simulink model "kalmannonlinear"  (R2019b)
settings: Solver=VariableStepAuto  StartTime=0.0  StopTime=10.0  RelTol=1e-3
libraries: sharedTrackingLibrary x2
settings Model: Creator=Bekircan Keceoglu  LastModifiedBy=Bekircan Keceoglu

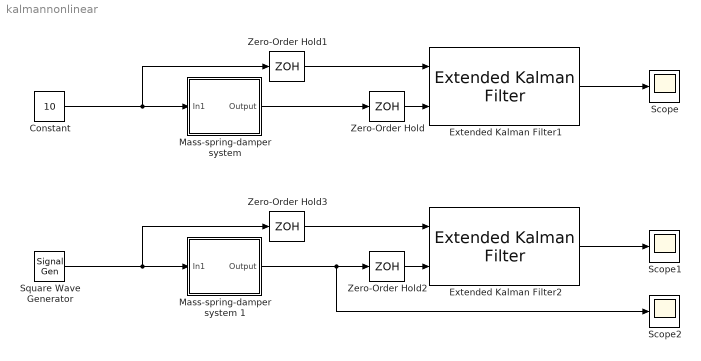
== system kalmannonlinear ==
  Constant : Constant  Value=10
  Extended Kalman Filter1 : sharedTrackingLibrary/Extended Kalman Filter  StateTransitionFcn=myStateTransitionFcn  HasStateTransitionJacobianFcn=off  HasAdditiveProcessNoise=Additive  ProcessNoise=1  HasTimeVaryingProcessNoise=off  HasStateTransitionFcnExtraArgument=1  InitialState=[0 0]  InitialStateCovariance=1  MeasurementFcn1=myMeasurementFcn  HasMeasurementJacobianFcn1=off  HasMeasurementEnablePort1=off  HasAdditiveMeasurementNoise1=Additive  MeasurementNoise1=1  HasTimeVaryingMeasurementNoise1=off  HasMeasurementFcnExtraArgument1=0  MeasurementFcn2=myMeasurementFcn  HasMeasurementJacobianFcn2=off  HasMeasurementEnablePort2=off  HasAdditiveMeasurementNoise2=Additive  MeasurementNoise2=1  HasTimeVaryingMeasurementNoise2=off  HasMeasurementFcnExtraArgument2=0  MeasurementFcn3=myMeasurementFcn  HasMeasurementJacobianFcn3=off  HasMeasurementEnablePort3=off  HasAdditiveMeasurementNoise3=Additive  MeasurementNoise3=1  HasTimeVaryingMeasurementNoise3=off  HasMeasurementFcnExtraArgument3=0  MeasurementFcn4=myMeasurementFcn  HasMeasurementJacobianFcn4=off  HasMeasurementEnablePort4=off  HasAdditiveMeasurementNoise4=Additive  MeasurementNoise4=1  HasTimeVaryingMeasurementNoise4=off  HasMeasurementFcnExtraArgument4=0  MeasurementFcn5=myMeasurementFcn  HasMeasurementJacobianFcn5=off  HasMeasurementEnablePort5=off  HasAdditiveMeasurementNoise5=Additive  MeasurementNoise5=1  HasTimeVaryingMeasurementNoise5=off  HasMeasurementFcnExtraArgument5=0  EnableMultirate=off  StateTransitionFcnSampleTime=1  MeasurementFcn1SampleTime=1  MeasurementFcn2SampleTime=1  MeasurementFcn3SampleTime=1  MeasurementFcn4SampleTime=1  MeasurementFcn5SampleTime=1  UseCurrentEstimator=on  OutputStateCovariance=off  DataType=double  SampleTime=10e-3  NumberOfMeasurements=1
      settings: SourceProductName=Control System Toolbox  SourceProductBaseCode=CT
  Extended Kalman Filter2 : sharedTrackingLibrary/Extended Kalman Filter  StateTransitionFcn=myStateTransitionFcn  HasStateTransitionJacobianFcn=off  HasAdditiveProcessNoise=Additive  ProcessNoise=1  HasTimeVaryingProcessNoise=off  HasStateTransitionFcnExtraArgument=1  InitialState=[0 0]  InitialStateCovariance=1  MeasurementFcn1=myMeasurementFcn  HasMeasurementJacobianFcn1=off  HasMeasurementEnablePort1=off  HasAdditiveMeasurementNoise1=Additive  MeasurementNoise1=1  HasTimeVaryingMeasurementNoise1=off  HasMeasurementFcnExtraArgument1=0  MeasurementFcn2=myMeasurementFcn  HasMeasurementJacobianFcn2=off  HasMeasurementEnablePort2=off  HasAdditiveMeasurementNoise2=Additive  MeasurementNoise2=1  HasTimeVaryingMeasurementNoise2=off  HasMeasurementFcnExtraArgument2=0  MeasurementFcn3=myMeasurementFcn  HasMeasurementJacobianFcn3=off  HasMeasurementEnablePort3=off  HasAdditiveMeasurementNoise3=Additive  MeasurementNoise3=1  HasTimeVaryingMeasurementNoise3=off  HasMeasurementFcnExtraArgument3=0  MeasurementFcn4=myMeasurementFcn  HasMeasurementJacobianFcn4=off  HasMeasurementEnablePort4=off  HasAdditiveMeasurementNoise4=Additive  MeasurementNoise4=1  HasTimeVaryingMeasurementNoise4=off  HasMeasurementFcnExtraArgument4=0  MeasurementFcn5=myMeasurementFcn  HasMeasurementJacobianFcn5=off  HasMeasurementEnablePort5=off  HasAdditiveMeasurementNoise5=Additive  MeasurementNoise5=1  HasTimeVaryingMeasurementNoise5=off  HasMeasurementFcnExtraArgument5=0  EnableMultirate=off  StateTransitionFcnSampleTime=1  MeasurementFcn1SampleTime=1  MeasurementFcn2SampleTime=1  MeasurementFcn3SampleTime=1  MeasurementFcn4SampleTime=1  MeasurementFcn5SampleTime=1  UseCurrentEstimator=on  OutputStateCovariance=off  DataType=double  SampleTime=10e-3  NumberOfMeasurements=1
      settings: SourceProductName=Control System Toolbox  SourceProductBaseCode=CT
  "Mass-spring-damper system " : Subsystem
  Mass-spring-damper system 1 : Subsystem
  Scope : Scope
  Scope1 : Scope
  Scope2 : Scope
  Square Wave Generator : SignalGenerator  WaveForm=square  Units=rad/sec
  Zero-Order Hold{,1..3} (4 alike) : ZeroOrderHold  SampleTime=10e-3
  wires:
  Constant/1 -> "Mass-spring-damper system "/1(In1), Zero-Order Hold1/1
  Zero-Order Hold1/1 -> Extended Kalman Filter1/1
  "Mass-spring-damper system "/1(Output) -> Zero-Order Hold/1
  Zero-Order Hold/1 -> Extended Kalman Filter1/2
  Extended Kalman Filter1/1 -> Scope/1
  Zero-Order Hold2/1 -> Extended Kalman Filter2/2
  Extended Kalman Filter2/1 -> Scope1/1
  Square Wave Generator/1 -> Mass-spring-damper system 1/1(In1), Zero-Order Hold3/1
  Mass-spring-damper system 1/1(Output) -> Scope2/1, Zero-Order Hold2/1
  Zero-Order Hold3/1 -> Extended Kalman Filter2/1

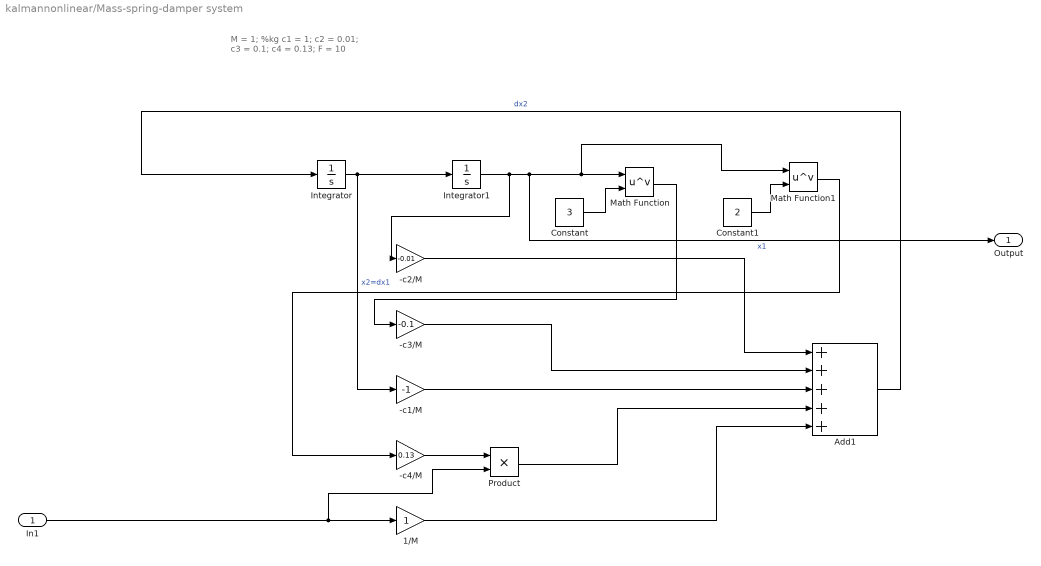
== system kalmannonlinear/Mass-spring-damper system  ==
  note: M  = 1; %kg
      | c1 = 1;
      | c2 = 0.01;
      | c3 = 0.1;
      | c4 = 0.13;
      | F  = 10
  In1 : Inport
  -c1/M : Gain  Gain=-1
  -c2/M : Gain  Gain=-0.01
  -c3/M : Gain  Gain=-0.1
  -c4/M : Gain  Gain=0.13
  1/M : Gain
  Add1 : Sum  Inputs=+++++
  Constant : Constant  Value=3
  Constant1 : Constant  Value=2
  Integrator : Integrator  InitialCondition=5
  Integrator1 : Integrator
  Math Function : Math  Operator=pow  SignedPower=off  SaturateOnIntegerOverflow=on
  Math Function1 : Math  Operator=pow  SignedPower=off  SaturateOnIntegerOverflow=on
  Product : Product
  Output : Outport
  wires:
  Integrator1/1 -> -c2/M/1, Output/1, Math Function1/1, Math Function/1  "x1"
  Math Function/1 -> -c3/M/1
  Constant/1 -> Math Function/2
  -c3/M/1 -> Add1/2
  Product/1 -> Add1/4
  -c1/M/1 -> Add1/3
  -c4/M/1 -> Product/1
  Math Function1/1 -> -c4/M/1
  Constant1/1 -> Math Function1/2
  -c2/M/1 -> Add1/1
  In1/1 -> Product/2, 1/M/1
  Integrator/1 -> -c1/M/1, Integrator1/1  "x2=dx1"
  Add1/1 -> Integrator/1  "dx2"
  1/M/1 -> Add1/5

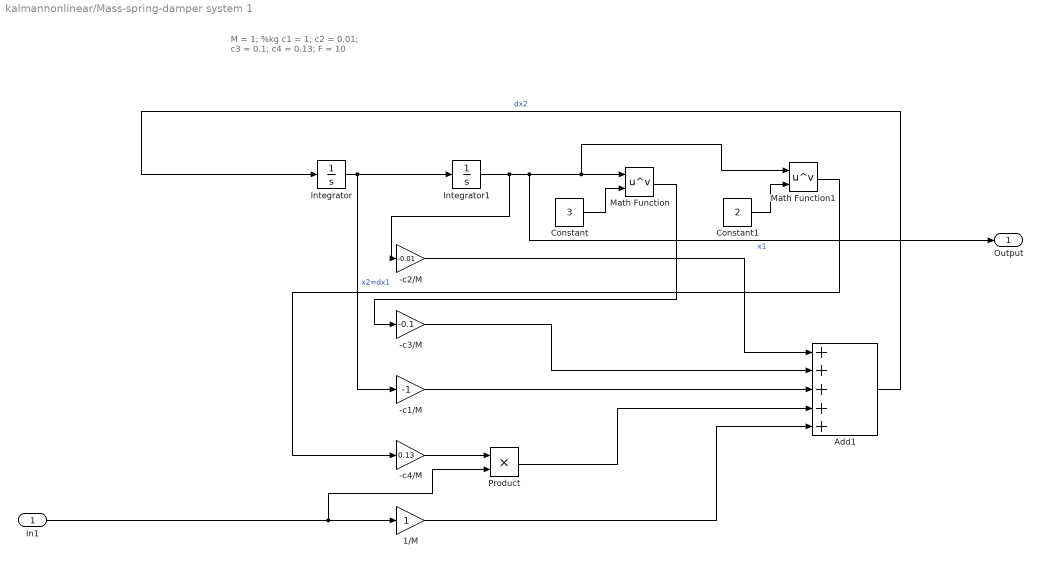
== system kalmannonlinear/Mass-spring-damper system 1 ==
  note: M  = 1; %kg
      | c1 = 1;
      | c2 = 0.01;
      | c3 = 0.1;
      | c4 = 0.13;
      | F  = 10
  In1 : Inport
  -c1/M : Gain  Gain=-1
  -c2/M : Gain  Gain=-0.01
  -c3/M : Gain  Gain=-0.1
  -c4/M : Gain  Gain=0.13
  1/M : Gain
  Add1 : Sum  Inputs=+++++
  Constant : Constant  Value=3
  Constant1 : Constant  Value=2
  Integrator : Integrator  InitialCondition=5
  Integrator1 : Integrator
  Math Function : Math  Operator=pow  SignedPower=off  SaturateOnIntegerOverflow=on
  Math Function1 : Math  Operator=pow  SignedPower=off  SaturateOnIntegerOverflow=on
  Product : Product
  Output : Outport
  wires:
  Integrator1/1 -> -c2/M/1, Output/1, Math Function1/1, Math Function/1  "x1"
  Math Function/1 -> -c3/M/1
  Constant/1 -> Math Function/2
  -c3/M/1 -> Add1/2
  Product/1 -> Add1/4
  -c1/M/1 -> Add1/3
  -c4/M/1 -> Product/1
  Math Function1/1 -> -c4/M/1
  Constant1/1 -> Math Function1/2
  -c2/M/1 -> Add1/1
  In1/1 -> Product/2, 1/M/1
  Integrator/1 -> -c1/M/1, Integrator1/1  "x2=dx1"
  Add1/1 -> Integrator/1  "dx2"
  1/M/1 -> Add1/5
